simulink model "Simulacion_Discretizada"  (R2020a)
settings: Solver=ode15s  StartTime=0.0  StopTime=20  MaxStep=1e-5  RelTol=1e-3
values from neighbouring files (symbols this model uses):
  alpha_cu = 3.9e-3    (= 0.0039)    [AnalisisDeEstabilidad.m]    (also in LTI_vs_LPV_vs_NL_realimentado.m; Modelo_linealizado.m)
  b_eq = b_m + b_l/(r^2)    (= 2.19444444444e-05)    [LTI_vs_LPV_vs_NL_realimentado.m]    (also in Modelo_linealizado.m)
  ba = 1    [parametros.m]
  C_ts = 0.818    [LTI_vs_LPV_vs_NL_realimentado.m]    (also in Modelo_linealizado.m)
  J_eq = J_m + J_l/(r^2)    (= 1.97847222222e-05)    [LTI_vs_LPV_vs_NL_realimentado.m]    (also in Modelo_linealizado.m)
  Ksa = 1    [parametros.m]
  L_d = 6.6/1000    (= 0.0066)    [Curvas_carc.m]    (also in LTI_vs_LPV_vs_NL_realimentado.m; Modelo_linealizado.m)
  L_ls = 0.8/1000    (= 0.0008)    [LTI_vs_LPV_vs_NL_realimentado.m]    (also in Modelo_linealizado.m)
  L_q = 5.8/1000    (= 0.0058)    [Curvas_carc.m]    (also in LTI_vs_LPV_vs_NL_realimentado.m; Modelo_linealizado.m)
  lambda_m = 0.01546    [Curvas_carc.m]    (also in LTI_vs_LPV_vs_NL_realimentado.m = 0.016; Modelo_linealizado.m = 0.016)
  P_p = 3    [Curvas_carc.m]    (also in LTI_vs_LPV_vs_NL_realimentado.m)
  r = 120    [AnalisisDeEstabilidad.m]    (also in LTI_vs_LPV_vs_NL_realimentado.m; Modelo_linealizado.m; parametros.m)
  R_sREF = R_sref    (= 1.02)    [LTI_vs_LPV_vs_NL_realimentado.m]
  R_ts_amb = 146.7    [LTI_vs_LPV_vs_NL_realimentado.m]    (also in Modelo_linealizado.m)
  Rdp = 3    [parametros.m]
  Rqp = 2    [parametros.m]
  sol = inv(A)*B    [Consigna_de_pos.m]
  sol2 = inv(A)*B    [Consigna_de_pos.m]
  T_amb = T_amb_o    (= 25)    [LTI_vs_LPV_vs_NL_realimentado.m]
  T_sREF = T_sref    (= 40)    [LTI_vs_LPV_vs_NL_realimentado.m]
undefined symbols (not defined in the file or in its folder): K_l, Ke_i, Ke_omega, Ke_theta, Ksia, sigbuilder_block, tau, Ts, V_max, w_n_i, w_n_pos, w_n_v, zit_i, zit_pos, zit_v
libraries: simulink x2
settings Model: Creator=matie  LastModifiedBy=matie

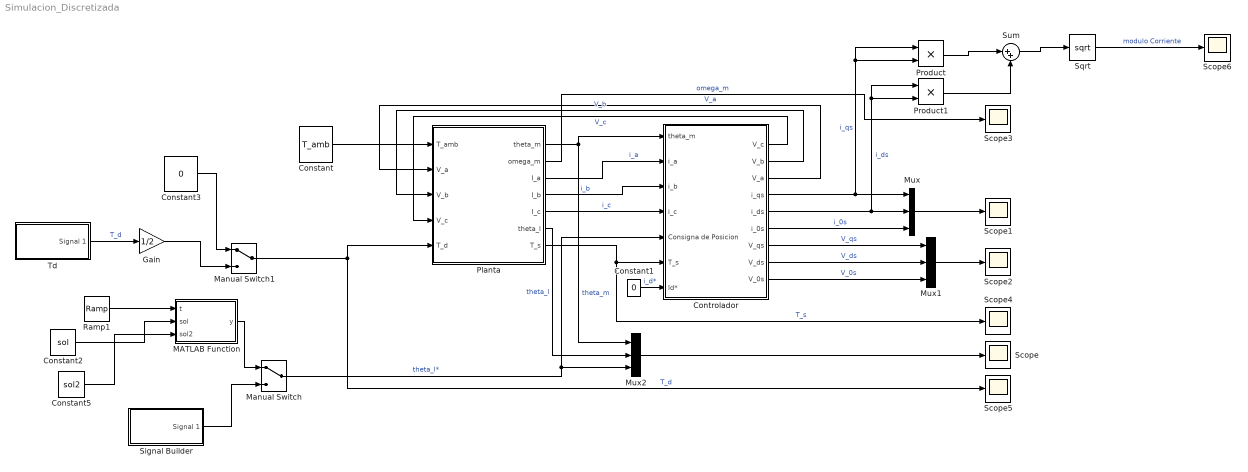
== system Simulacion_Discretizada ==
  Constant : Constant  Value=T_amb  VectorParams1D=off  SampleTime=-1
  Constant1 : Constant  Value=0
  Constant2 : Constant  Value=sol  VectorParams1D=off
  Constant3 : Constant  Value=0  VectorParams1D=off  SampleTime=-1
  Constant5 : Constant  Value=sol2  VectorParams1D=off
  Controlador : Subsystem
  Gain : Gain  Gain=1/2
  MATLAB Function : MATLAB Function  TreatAsAtomicUnit=on
  Manual Switch : ManualSwitch
  Manual Switch1 : ManualSwitch
  Mux : Mux  Inputs=3
  Mux1 : Mux  Inputs=3
  Mux2 : Mux  Inputs=3
  Planta : Subsystem
  Product : Product
  Product1 : Product
  Ramp1 : simulink/Sources/Ramp  slope=1  start=0  InitialOutput=0
  Scope{,1..6} (7 alike) : Scope
  Signal Builder : Subsystem  Tag=STV Subsys  LoadFcn=sigbuilder_block('load');  StartFcn=sigbuilder_block('start');  StopFcn=sigbuilder_block('stop');  ClipboardFcn=sigbuilder_block('clipboard');  mask(Sigbuilder block){tuvar=[0:10]}
      mask help: Simulink:masks:SigbuilderBlock_MD
      mask init:
      | if ~strcmp(get_param(bdroot(gcbh),'SimulationStatus'),'stopped') tuvar = sigbuilder_block('maskInit'); end
      settings: CopyFcn=sigbuilder_block('copy');  DeleteFcn=sigbuilder_block('delete');  ModelCloseFcn=sigbuilder_block('modelClose');  PreSaveFcn=sigbuilder_block('preSave');  PauseFcn=sigbuilder_block('pause');  ContinueFcn=sigbuilder_block('continue');  NameChangeFcn=sigbuilder_block('namechange');  OpenFcn=sigbuilder_block('open',[437.6 199.2 550.4 400 ]);  CloseFcn=sigbuilder_block('close');
      mask Display: plot(0, 0, 100, 100,[2, 2, 32, 32, 2], [68, 8, 8, 68, 68],[32, 2], [38, 38], [32, 19, 2],[53, 60, 44], [32, 17, 17, 2],[16, 16, 31, 31]);txt = getActiveGroup(gcbh);text(2, 100, txt,'verticalAlignment', 'top');
  Sqrt : Sqrt  SaturateOnIntegerOverflow=on
  Sum : Sum  Inputs=|++
  Td : Subsystem  Tag=STV Subsys  LoadFcn=sigbuilder_block('load');  StartFcn=sigbuilder_block('start');  StopFcn=sigbuilder_block('stop');  ClipboardFcn=sigbuilder_block('clipboard');  mask(Sigbuilder block){tuvar=[0:10]}
      mask help: Simulink:masks:SigbuilderBlock_MD
      mask init:
      | if ~strcmp(get_param(bdroot(gcbh),'SimulationStatus'),'stopped') tuvar = sigbuilder_block('maskInit'); end
      settings: CopyFcn=sigbuilder_block('copy');  DeleteFcn=sigbuilder_block('delete');  ModelCloseFcn=sigbuilder_block('modelClose');  PreSaveFcn=sigbuilder_block('preSave');  PauseFcn=sigbuilder_block('pause');  ContinueFcn=sigbuilder_block('continue');  NameChangeFcn=sigbuilder_block('namechange');  OpenFcn=sigbuilder_block('open',[437.6 199.2 550.4 400 ]);  CloseFcn=sigbuilder_block('close');
      mask Display: plot(0, 0, 100, 100,[2, 2, 32, 32, 2], [68, 8, 8, 68, 68],[32, 2], [38, 38], [32, 19, 2],[53, 60, 44], [32, 17, 17, 2],[16, 16, 31, 31]);txt = getActiveGroup(gcbh);text(2, 100, txt,'verticalAlignment', 'top');
  wires:
  Constant/1 -> Planta/1(T_amb)
  Planta/1(theta_m) -> Controlador/1(theta_m), Mux2/1  "theta_m"
  Planta/2(omega_m) -> Scope3/1  "omega_m"
  Planta/3(I_a) -> Controlador/2(i_a)  "i_a"
  Planta/4(I_b) -> Controlador/3(i_b)  "i_b"
  Planta/5(I_c) -> Controlador/4(i_c)  "i_c"
  Controlador/1(V_c) -> Planta/4(V_c)  "V_c"
  Controlador/2(V_b) -> Planta/3(V_b)  "V_b"
  Controlador/3(V_a) -> Planta/2(V_a)  "V_a"
  Constant1/1 -> Controlador/7(Id*)  "i_d*"
  Planta/7(T_s) -> Scope4/1, Controlador/6(T_s)  "T_s"
  Controlador/4(i_qs) -> Product/2, Product/1, Mux/1  "i_qs"
  Controlador/5(i_ds) -> Product1/2, Product1/1, Mux/2  "i_ds"
  Controlador/6(i_0s) -> Mux/3  "i_0s"
  Controlador/7(V_qs) -> Mux1/1  "V_qs"
  Controlador/8(V_ds) -> Mux1/2  "V_ds"
  Controlador/9(V_0s) -> Mux1/3  "V_0s"
  Planta/6(theta_l) -> Mux2/2  "theta_l"
  Manual Switch1/1 -> Planta/5(T_d), Scope5/1  "T_d"
  Manual Switch/1 -> Controlador/5(Consigna de Posicion), Mux2/3  "theta_l*"
  Mux2/1 -> Scope/1
  Mux/1 -> Scope1/1
  Mux1/1 -> Scope2/1
  Constant5/1 -> MATLAB Function/3(sol2)
  Ramp1/1 -> MATLAB Function/1(t)
  Constant2/1 -> MATLAB Function/2(sol)
  MATLAB Function/1(y) -> Manual Switch/1
  Signal Builder/1(Signal 1) -> Manual Switch/2
  Td/1(Signal 1) -> Gain/1  "T_d"
  Constant3/1 -> Manual Switch1/1
  Product/1 -> Sum/1
  Product1/1 -> Sum/2
  Sum/1 -> Sqrt/1
  Sqrt/1 -> Scope6/1  "modulo Corriente"
  Gain/1 -> Manual Switch1/2

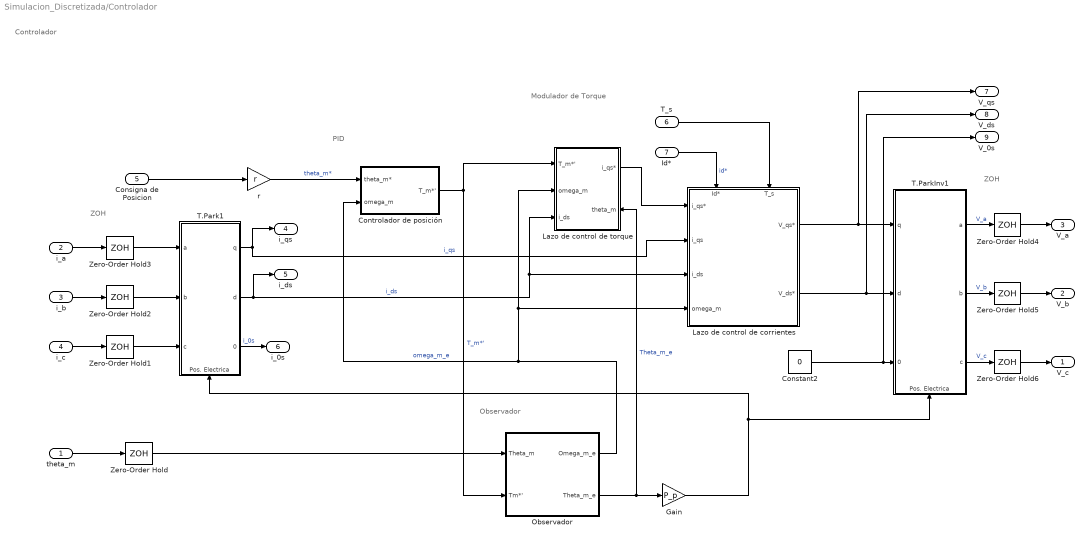
== system Simulacion_Discretizada/Controlador ==
  note: ZOH
  note: ZOH
  note: Observador
  note: Controlador
  note: PID
  note: Modulador de Torque
  theta_m : Inport
  i_a : Inport  Port=2
  i_b : Inport  Port=3
  i_c : Inport  Port=4
  Consigna de Posicion : Inport  Port=5
  T_s : Inport  Port=6
  Id* : Inport  Port=7
  Constant2 : Constant  Value=0
  Controlador de posición : Subsystem
  Gain : Gain  Gain=P_p
  Lazo de control de corrientes : Subsystem
      settings: PortSchema="{\"entries\":[{\"content\":{\"sides\":[{\"content\":{\"connectorIds\":[\"In1\",\"In2\",\"In3\",\"In4\"]},\"type\":\"ConnectorPlacement.EquallySpacedRectSide\",\"uuid\":\"8590a798-b272-4dda-94d3-b02bfe7981cd\"},{\"content\":{\"connectorIds\":[\"Out1\",\"Out2\"],\"side\":\"RIGHT\"},\"type\":\"ConnectorPlacement.EquallySpacedRectSide\",\"uuid\":\"79f7ba4f-ca3d-417b-a956-e8ff79666446\"},{\"content\":{\"connectorIds\":[\"In5\",\"In6\"],\"side\":\"TOP\"},\"type\":\"ConnectorPlacement.EquallySpacedRectSide\",\"uuid\":\"c783970f-a0cd-49ae-b0d9-9eb7b782510c\"}]},\"type\":\"ConnectorPlacement.EquallySpacedConnector\",\"uuid\":\"7f007081-b507-4644-8a4e-ff370ccc3754\"}],\"packageUris\":[\"http://schema.mathworks.com/mf0/Connector/19700101\"],\"version\":\"1.0\"}"
  Lazo de control de torque : Subsystem
      settings: PortSchema="{\"entries\":[{\"content\":{\"sides\":[{\"content\":{\"connectorIds\":[\"In1\",\"In2\",\"In3\"]},\"type\":\"ConnectorPlacement.EquallySpacedRectSide\",\"uuid\":\"ab0e8616-8d3e-4cd7-8423-bd93729455f6\"},{\"content\":{\"connectorIds\":[\"Out1\",\"In4\"],\"side\":\"RIGHT\"},\"type\":\"ConnectorPlacement.EquallySpacedRectSide\",\"uuid\":\"bacb25e2-23a7-49b0-9cd8-46522174ac61\"},{\"content\":{\"connectorIds\":[],\"side\":\"TOP\"},\"type\":\"ConnectorPlacement.EquallySpacedRectSide\",\"uuid\":\"92980fe9-d82b-422b-ba0e-4e399ce43552\"},{\"content\":{\"connectorIds\":[],\"side\":\"BOTTOM\"},\"type\":\"ConnectorPlacement.EquallySpacedRectSide\",\"uuid\":\"d03b3e30-9585-41dd-826f-10e3a5c14235\"}]},\"type\":\"ConnectorPlacement.EquallySpacedConnector\",\"uuid\":\"7c3e8c07-5c99-45fd-a37d-868b0a52132c\"}],\"packageUris\":[\"http://schema.mathworks.com/mf0/Connector/19700101\"],\"version\":\"1.0\"}"
  Observador : Subsystem
  T.Park1 : Subsystem
      settings: PortSchema="{\"entries\":[{\"content\":{\"sides\":[{\"content\":{\"connectorIds\":[\"In1\",\"In2\",\"In3\"]},\"type\":\"ConnectorPlacement.EquallySpacedRectSide\",\"uuid\":\"2bfbe7ef-652a-4797-b13c-b84c243bd68c\"},{\"content\":{\"connectorIds\":[\"Out1\",\"Out2\",\"Out3\"],\"side\":\"RIGHT\"},\"type\":\"ConnectorPlacement.EquallySpacedRectSide\",\"uuid\":\"075def0e-c436-44dc-ba25-82cf6ffae869\"},{\"content\":{\"connectorIds\":[\"In4\"],\"side\":\"TOP\"},\"type\":\"ConnectorPlacement.EquallySpacedRectSide\",\"uuid\":\"95d81334-e332-4f04-a2cb-c4692f91809c\"},{\"content\":{\"connectorIds\":[],\"side\":\"BOTTOM\"},\"type\":\"ConnectorPlacement.EquallySpacedRectSide\",\"uuid\":\"85b95360-e43d-49d1-a18f-690334b045e6\"}]},\"type\":\"ConnectorPlacement.EquallySpacedConnector\",\"uuid\":\"b90f9cad-0277-459c-bcac-17172872a787\"}],\"packageUris\":[\"http://schema.mathworks.com/mf0/Connector/19700101\"],\"version\":\"1.0\"}"
  T.ParkInv1 : Subsystem
      settings: PortSchema="{\"entries\":[{\"content\":{\"sides\":[{\"content\":{\"connectorIds\":[\"In1\",\"In2\",\"In3\"]},\"type\":\"ConnectorPlacement.EquallySpacedRectSide\",\"uuid\":\"aef3590a-5fc0-4a95-8f41-1fc79c0f3fe7\"},{\"content\":{\"connectorIds\":[\"Out1\",\"Out2\",\"Out3\"],\"side\":\"RIGHT\"},\"type\":\"ConnectorPlacement.EquallySpacedRectSide\",\"uuid\":\"4e7c387b-9bca-48cc-a151-2357bd6b7b1d\"},{\"content\":{\"connectorIds\":[],\"side\":\"TOP\"},\"type\":\"ConnectorPlacement.EquallySpacedRectSide\",\"uuid\":\"1231932f-f9d3-49e6-b404-2af91cb220c6\"},{\"content\":{\"connectorIds\":[\"In4\"],\"side\":\"BOTTOM\"},\"type\":\"ConnectorPlacement.EquallySpacedRectSide\",\"uuid\":\"5c8d0cfe-c367-499e-bd37-95f7c8af20a1\"}]},\"type\":\"ConnectorPlacement.EquallySpacedConnector\",\"uuid\":\"48e39a78-817d-4753-b518-4d689d2c1635\"}],\"packageUris\":[\"http://schema.mathworks.com/mf0/Connector/19700101\"],\"version\":\"1.0\"}"
  Zero-Order Hold{,1..6} (7 alike) : ZeroOrderHold  SampleTime=Ts
  r : Gain  Gain=r
  V_c : Outport
  V_b : Outport  Port=2
  V_a : Outport  Port=3
  i_qs : Outport  Port=4
  i_ds : Outport  Port=5
  i_0s : Outport  Port=6
  V_qs : Outport  Port=7
  V_ds : Outport  Port=8
  V_0s : Outport  Port=9
  wires:
  i_b/1 -> Zero-Order Hold2/1
  i_a/1 -> Zero-Order Hold3/1
  i_c/1 -> Zero-Order Hold1/1
  T.Park1/1(0) -> i_0s/1  "i_0s"
  T.Park1/2(d) -> Lazo de control de torque/3(i_ds), Lazo de control de corrientes/3(i_ds), i_ds/1  "i_ds"
  T_s/1 -> Lazo de control de corrientes/6(T_s)
  Observador/1(Omega_m_e) -> Controlador de posición/2(omega_m), Lazo de control de torque/2(omega_m), Lazo de control de corrientes/4(omega_m)  "omega_m_e"
  T.Park1/3(q) -> i_qs/1, Lazo de control de corrientes/2(i_qs)  "i_qs"
  Gain/1 -> T.Park1/4(Pos. Electrica), T.ParkInv1/4(Pos. Electrica)
  Controlador de posición/1(T_m*') -> Lazo de control de torque/1(T_m*'), Observador/2(Tm*')  "T_m*'"
  Consigna de Posicion/1 -> r/1
  T.ParkInv1/3(c) -> Zero-Order Hold6/1  "V_c"
  T.ParkInv1/2(b) -> Zero-Order Hold5/1  "V_b"
  T.ParkInv1/1(a) -> Zero-Order Hold4/1  "V_a"
  Constant2/1 -> V_0s/1, T.ParkInv1/3(0)
  theta_m/1 -> Zero-Order Hold/1
  Observador/2(Theta_m_e) -> Gain/1, Lazo de control de torque/4(theta_m)  "Theta_m_e"
  Lazo de control de corrientes/2(V_ds*) -> V_ds/1, T.ParkInv1/2(d)
  Lazo de control de corrientes/1(V_qs*) -> V_qs/1, T.ParkInv1/1(q)
  Lazo de control de torque/1(i_qs*) -> Lazo de control de corrientes/1(i_qs*)
  Id*/1 -> Lazo de control de corrientes/5(Id*)  "id*"
  r/1 -> Controlador de posición/1(theta_m*)  "theta_m*"
  Zero-Order Hold/1 -> Observador/1(Theta_m)
  Zero-Order Hold1/1 -> T.Park1/1(c)
  Zero-Order Hold2/1 -> T.Park1/2(b)
  Zero-Order Hold3/1 -> T.Park1/3(a)
  Zero-Order Hold4/1 -> V_a/1
  Zero-Order Hold5/1 -> V_b/1
  Zero-Order Hold6/1 -> V_c/1

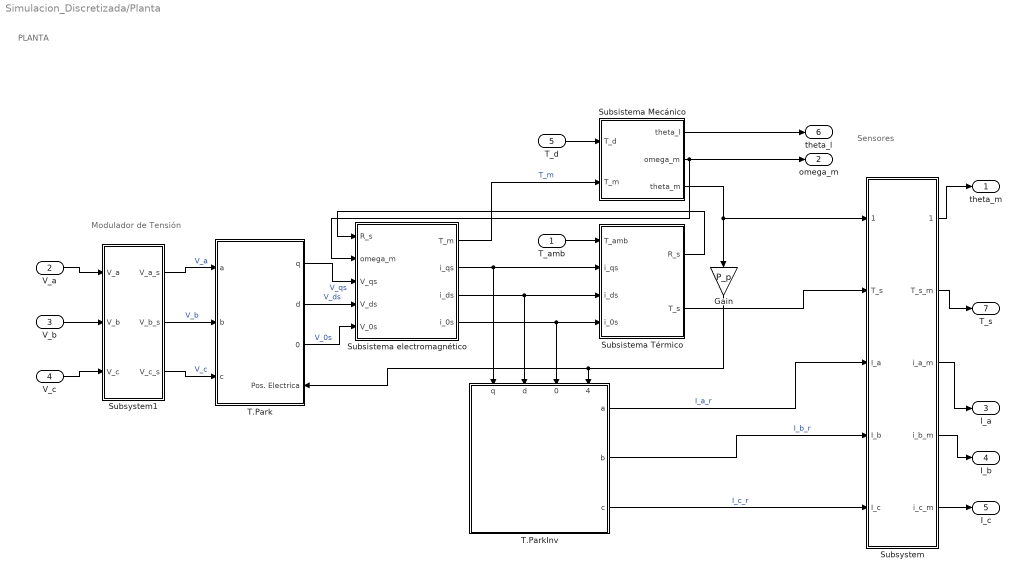
== system Simulacion_Discretizada/Planta ==
  note: PLANTA
  note: Sensores
  note: Modulador de
      | Tensión
  T_amb : Inport
  V_a : Inport  Port=2
  V_b : Inport  Port=3
  V_c : Inport  Port=4
  T_d : Inport  Port=5
  "\tSubsistema Térmico" : Subsystem
  Gain : Gain  Gain=P_p
  Subsistema Mecánico : Subsystem
  Subsistema electromagnético : Subsystem
  Subsystem : Subsystem
  Subsystem1 : Subsystem
  T.Park : Subsystem
      settings: PortSchema="{\"entries\":[{\"content\":{\"sides\":[{\"content\":{\"connectorIds\":[\"In1\",\"In2\",\"In3\"]},\"type\":\"ConnectorPlacement.EquallySpacedRectSide\",\"uuid\":\"2bfbe7ef-652a-4797-b13c-b84c243bd68c\"},{\"content\":{\"connectorIds\":[\"Out1\",\"Out2\",\"Out3\",\"In4\"],\"side\":\"RIGHT\"},\"type\":\"ConnectorPlacement.EquallySpacedRectSide\",\"uuid\":\"075def0e-c436-44dc-ba25-82cf6ffae869\"},{\"content\":{\"connectorIds\":[],\"side\":\"TOP\"},\"type\":\"ConnectorPlacement.EquallySpacedRectSide\",\"uuid\":\"95d81334-e332-4f04-a2cb-c4692f91809c\"}]},\"type\":\"ConnectorPlacement.EquallySpacedConnector\",\"uuid\":\"b90f9cad-0277-459c-bcac-17172872a787\"}],\"packageUris\":[\"http://schema.mathworks.com/mf0/Connector/19700101\"],\"version\":\"1.0\"}"
  T.ParkInv : Subsystem
      settings: PortSchema="{\"entries\":[{\"content\":{\"sides\":[{\"content\":{\"connectorIds\":[\"In1\",\"In2\",\"In3\",\"In4\"]},\"type\":\"ConnectorPlacement.EquallySpacedRectSide\",\"uuid\":\"aef3590a-5fc0-4a95-8f41-1fc79c0f3fe7\"},{\"content\":{\"connectorIds\":[],\"side\":\"RIGHT\"},\"type\":\"ConnectorPlacement.EquallySpacedRectSide\",\"uuid\":\"4e7c387b-9bca-48cc-a151-2357bd6b7b1d\"},{\"content\":{\"connectorIds\":[],\"side\":\"TOP\"},\"type\":\"ConnectorPlacement.EquallySpacedRectSide\",\"uuid\":\"1231932f-f9d3-49e6-b404-2af91cb220c6\"},{\"content\":{\"connectorIds\":[\"Out1\",\"Out2\",\"Out3\"],\"side\":\"BOTTOM\"},\"type\":\"ConnectorPlacement.EquallySpacedRectSide\",\"uuid\":\"4f29e626-7677-496e-bb82-59a3ecbc7a95\"}]},\"type\":\"ConnectorPlacement.EquallySpacedConnector\",\"uuid\":\"48e39a78-817d-4753-b518-4d689d2c1635\"}],\"packageUris\":[\"http://schema.mathworks.com/mf0/Connector/19700101\"],\"version\":\"1.0\"}"
  theta_m : Outport
  omega_m : Outport  Port=2
  I_a : Outport  Port=3
  I_b : Outport  Port=4
  I_c : Outport  Port=5
  theta_l : Outport  Port=6
  T_s : Outport  Port=7
  wires:
  Subsistema Mecánico/3(theta_m) -> Subsystem/1(theta_m), Gain/1
  Gain/1 -> T.Park/4(Pos. Electrica), T.ParkInv/4(Pos. Electrica)
  T.Park/1(q) -> Subsistema electromagnético/3(V_qs)  "V_qs"
  Subsistema Mecánico/2(omega_m) -> Subsistema electromagnético/2(omega_m), omega_m/1
  Subsistema electromagnético/2(i_qs) -> "\tSubsistema Térmico"/2(i_qs), T.ParkInv/1(q)
  Subsistema electromagnético/1(T_m) -> Subsistema Mecánico/2(T_m)  "T_m"
  Subsistema electromagnético/4(i_0s) -> "\tSubsistema Térmico"/4(i_0s), T.ParkInv/3(0)
  Subsistema electromagnético/3(i_ds) -> "\tSubsistema Térmico"/3(i_ds), T.ParkInv/2(d)
  Subsistema Mecánico/1(theta_l) -> theta_l/1
  T.Park/3(0) -> Subsistema electromagnético/5(V_0s)  "V_0s"
  T.Park/2(d) -> Subsistema electromagnético/4(V_ds)  "V_ds"
  T_d/1 -> Subsistema Mecánico/1(T_d)
  T_amb/1 -> "\tSubsistema Térmico"/1(T_amb)
  "\tSubsistema Térmico"/1(R_s) -> Subsistema electromagnético/1(R_s)
  "\tSubsistema Térmico"/2(T_s) -> Subsystem/2(T_s)
  T.ParkInv/1(a) -> Subsystem/3(I_a)  "I_a_r"
  T.ParkInv/2(b) -> Subsystem/4(I_b)  "I_b_r"
  T.ParkInv/3(c) -> Subsystem/5(I_c)  "I_c_r"
  Subsystem/1(theta_m_m) -> theta_m/1
  Subsystem/2(T_s_m) -> T_s/1
  Subsystem/3(i_a_m) -> I_a/1
  Subsystem/4(i_b_m) -> I_b/1
  Subsystem/5(i_c_m) -> I_c/1
  V_a/1 -> Subsystem1/1(V_a)
  V_b/1 -> Subsystem1/2(V_b)
  V_c/1 -> Subsystem1/3(V_c)
  Subsystem1/1(V_a_s) -> T.Park/1(a)  "V_a"
  Subsystem1/2(V_b_s) -> T.Park/2(b)  "V_b"
  Subsystem1/3(V_c_s) -> T.Park/3(c)  "V_c"

== system Simulacion_Discretizada/Signal Builder ==
  Demux : Demux  Tag=STV Demux  Outputs=1
      settings: DisplayOption=none
  FromWs : FromWorkspace  Tag=STV FromWs  VariableName=tuvar
      SigBuilderData=|
      | common.afterFinalStr = 'Extrapolate'
      | common.sampleTime = 0
      | dataSet.timeRange = [0 20]
      | dataSet.name = 'Group 1'
      | sbobj.Groups.Name = 'Group 1'
      | sbobj.Groups.Signals.Name = 'Signal 1'
      | sbobj.Groups.Signals.XData = [0 1 6 11 16 20]
      | sbobj.Groups.Signals.YData = [0 0 6.28318530718 6.28318530718 0 0]
      | sbobj.Groups.TimeRange = [0 20]
  Signal 1 : Outport  Tag=STV Outport
  wires:
  Demux/1 -> Signal 1/1
  FromWs/1 -> Demux/1

== system Simulacion_Discretizada/Td ==
  Demux : Demux  Tag=STV Demux  Outputs=1
      settings: DisplayOption=none
  FromWs : FromWorkspace  Tag=STV FromWs  VariableName=tuvar
      SigBuilderData=|
      | common.afterFinalStr = 'Extrapolate'
      | common.sampleTime = 0
      | dataSet.timeRange = [0 20]
      | dataSet.name = 'Group 1'
      | sbobj.Groups.Name = 'Group 1'
      | sbobj.Groups.Signals.Name = 'Signal 1'
      | sbobj.Groups.Signals.XData = [0 6.5 6.5 8.5 8.5 10.5 10.5 20]
      | sbobj.Groups.Signals.YData = [0 0 5 5 -5 -5 0 0]
      | sbobj.Groups.TimeRange = [0 20]
  Signal 1 : Outport  Tag=STV Outport
  wires:
  Demux/1 -> Signal 1/1
  FromWs/1 -> Demux/1

== system Simulacion_Discretizada/Controlador/Controlador de posición ==
  theta_m* : Inport
  omega_m : Inport  Port=2
  Constant2 : Constant  Value=sol  VectorParams1D=off
  Constant5 : Constant  Value=sol2  VectorParams1D=off
  Derivative : Derivative  CoefficientInTFapproximation=0
  Gain : Gain  Gain=r
  Manual Switch : ManualSwitch
  Ramp : simulink/Sources/Ramp  slope=1  start=0  InitialOutput=0
  Subsystem : Subsystem
  consigna_velocidad : MATLAB Function  TreatAsAtomicUnit=on
  T_m*' : Outport
  wires:
  theta_m*/1 -> Derivative/1
  Constant5/1 -> consigna_velocidad/3(sol2)
  Constant2/1 -> consigna_velocidad/2(sol)
  Derivative/1 -> Manual Switch/2  "omega_m*"
  consigna_velocidad/1(y) -> Gain/1
  Gain/1 -> Manual Switch/1
  Ramp/1 -> consigna_velocidad/1(t)
  Manual Switch/1 -> Subsystem/1(omega_m*)  "omega_m*"
  omega_m/1 -> Subsystem/2(omega_m)
  Subsystem/1(T_m*') -> T_m*'/1

== system Simulacion_Discretizada/Controlador/Lazo de control de corrientes ==
  i_qs* : Inport
  i_qs : Inport  Port=2
  i_ds : Inport  Port=3
  omega_m : Inport  Port=4
  Id* : Inport  Port=5
  T_s : Inport  Port=6
  Control de I_ds : Subsystem
      settings: PortSchema="{\"entries\":[{\"content\":{\"sides\":[{\"content\":{\"connectorIds\":[\"In1\",\"In2\",\"In3\",\"In4\"]},\"type\":\"ConnectorPlacement.EquallySpacedRectSide\",\"uuid\":\"ffce1851-57e2-41df-aed0-a87e2179134d\"},{\"content\":{\"connectorIds\":[\"Out1\"],\"side\":\"RIGHT\"},\"type\":\"ConnectorPlacement.EquallySpacedRectSide\",\"uuid\":\"747f8c9d-35f1-4917-b439-3fa2ce1f796d\"},{\"content\":{\"connectorIds\":[],\"side\":\"TOP\"},\"type\":\"ConnectorPlacement.EquallySpacedRectSide\",\"uuid\":\"8177f07d-0fa6-4905-a4da-67659c71ef29\"},{\"content\":{\"connectorIds\":[\"In5\"],\"side\":\"BOTTOM\"},\"type\":\"ConnectorPlacement.EquallySpacedRectSide\",\"uuid\":\"6dd9ac8a-27c9-4038-bd4e-8ef4f6a79f96\"}]},\"type\":\"ConnectorPlacement.EquallySpacedConnector\",\"uuid\":\"e8499173-6965-4bf7-863b-b1df3b035aa5\"}],\"packageUris\":[\"http://schema.mathworks.com/mf0/Connector/19700101\"],\"version\":\"1.0\"}"
  Control de I_qs : Subsystem
      settings: PortSchema="{\"entries\":[{\"content\":{\"sides\":[{\"content\":{\"connectorIds\":[\"In1\",\"In2\",\"In3\",\"In4\"]},\"type\":\"ConnectorPlacement.EquallySpacedRectSide\",\"uuid\":\"ffce1851-57e2-41df-aed0-a87e2179134d\"},{\"content\":{\"connectorIds\":[\"Out1\"],\"side\":\"RIGHT\"},\"type\":\"ConnectorPlacement.EquallySpacedRectSide\",\"uuid\":\"747f8c9d-35f1-4917-b439-3fa2ce1f796d\"},{\"content\":{\"connectorIds\":[\"In5\"],\"side\":\"TOP\"},\"type\":\"ConnectorPlacement.EquallySpacedRectSide\",\"uuid\":\"8177f07d-0fa6-4905-a4da-67659c71ef29\"}]},\"type\":\"ConnectorPlacement.EquallySpacedConnector\",\"uuid\":\"e8499173-6965-4bf7-863b-b1df3b035aa5\"}],\"packageUris\":[\"http://schema.mathworks.com/mf0/Connector/19700101\"],\"version\":\"1.0\"}"
  Evolución R_s : Subsystem
  Gain10 : Gain  Gain=P_p
  V_qs* : Outport
  V_ds* : Outport  Port=2
  wires:
  Gain10/1 -> Control de I_qs/1(omega_e), Control de I_ds/4(omega_e)
  i_qs*/1 -> Control de I_qs/5(i_qs*)
  i_ds/1 -> Control de I_qs/3(i_ds), Control de I_ds/1(i_ds)
  Control de I_qs/1(V_qs*) -> V_qs*/1
  i_qs/1 -> Control de I_qs/4(i_qs), Control de I_ds/2(i_qs)
  T_s/1 -> Evolución R_s/1(T_s)
  Control de I_ds/1(V_ds*) -> V_ds*/1
  omega_m/1 -> Gain10/1
  Id*/1 -> Control de I_ds/5(i_ds*)
  Evolución R_s/1(R_s) -> Control de I_ds/3(R_s), Control de I_qs/2(R_s)

== system Simulacion_Discretizada/Controlador/Lazo de control de torque ==
  note: Linealización por realimentación no lineal
  note: T_m*
  T_m*' : Inport
  omega_m : Inport  Port=2
  i_ds : Inport  Port=3
  theta_m : Inport  Port=4
  1/r : Gain  Gain=1/r
  Constant3 : Constant  Value=lambda_m
  Divide : Product  Inputs=*/
  Gain3 : Gain  Gain=b_eq
  Gain4 : Gain  Gain=L_d-L_q
  Gain5 : Gain  Gain=3*P_p/2
  Kl/r : Gain  Gain=K_l/r
  Sum11 : Sum  Inputs=|+++
  Sum12 : Sum  Inputs=|++
  Trigonometric Function2 : Trigonometry
  i_qs* : Outport
  wires:
  i_ds/1 -> Gain4/1
  Gain4/1 -> Sum12/2
  Gain3/1 -> Sum11/3
  omega_m/1 -> Gain3/1
  Sum11/1 -> Divide/1  "T_m*"
  Constant3/1 -> Sum12/1
  Gain5/1 -> Divide/2
  Sum12/1 -> Gain5/1
  Divide/1 -> i_qs*/1  "i_qs*"
  T_m*'/1 -> Sum11/2
  Trigonometric Function2/1 -> Kl/r/1
  1/r/1 -> Trigonometric Function2/1
  Kl/r/1 -> Sum11/1
  theta_m/1 -> 1/r/1

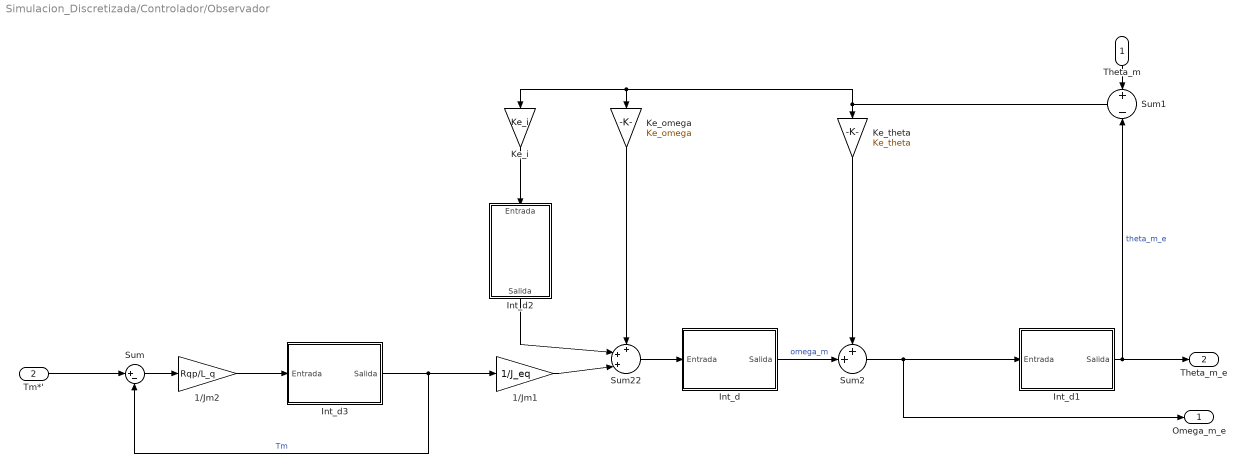
== system Simulacion_Discretizada/Controlador/Observador ==
  Theta_m : Inport
  Tm*' : Inport  Port=2
  1/Jm1 : Gain  Gain=1/J_eq
  1/Jm2 : Gain  Gain=Rqp/L_q
  Int_d : Subsystem
  Int_d1 : Subsystem
  Int_d2 : Subsystem
  Int_d3 : Subsystem
  Ke_i : Gain  Gain=Ke_i
  Ke_omega : Gain  Gain=Ke_omega
  Ke_theta : Gain  Gain=Ke_theta
  Sum : Sum  Inputs=|+-
  Sum1 : Sum  Inputs=+-
  Sum2 : Sum  Inputs=++|
  Sum22 : Sum  Inputs=+++|
  Omega_m_e : Outport
  Theta_m_e : Outport  Port=2
  wires:
  Ke_omega/1 -> Sum22/1
  Sum2/1 -> Int_d1/1(Entrada), Omega_m_e/1
  Ke_theta/1 -> Sum2/1
  1/Jm1/1 -> Sum22/3
  Theta_m/1 -> Sum1/1
  Tm*'/1 -> Sum/1
  Int_d3/1(Salida) -> 1/Jm1/1, Sum/2  "Tm"
  Int_d2/1(Salida) -> Sum22/2
  Sum1/1 -> Ke_i/1, Ke_omega/1, Ke_theta/1
  Ke_i/1 -> Int_d2/1(Entrada)
  Sum22/1 -> Int_d/1(Entrada)
  Int_d/1(Salida) -> Sum2/2  "omega_m"
  Int_d1/1(Salida) -> Theta_m_e/1, Sum1/2  "theta_m_e"
  Sum/1 -> 1/Jm2/1
  1/Jm2/1 -> Int_d3/1(Entrada)

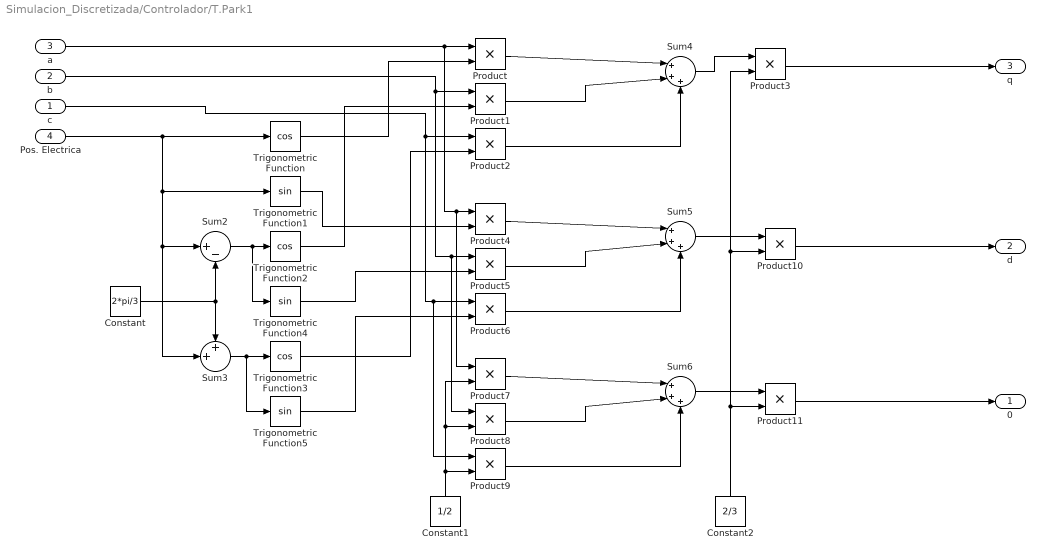
== system Simulacion_Discretizada/Controlador/T.Park1 ==
  c : Inport
  b : Inport  Port=2
  a : Inport  Port=3
  Pos. Electrica : Inport  Port=4
  Constant : Constant  Value=2*pi/3
  Constant1 : Constant  Value=1/2
  Constant2 : Constant  Value=2/3
  Product{,1..11} (12 alike) : Product
  Sum2 : Sum  Inputs=|+-
  Sum3 : Sum  Inputs=++|
  Sum4 : Sum  Inputs=|+++
  Sum5 : Sum  Inputs=|+++
  Sum6 : Sum  Inputs=|+++
  Trigonometric Function : Trigonometry  Operator=cos
  Trigonometric Function1 : Trigonometry
  Trigonometric Function2 : Trigonometry  Operator=cos
  Trigonometric Function3 : Trigonometry  Operator=cos
  Trigonometric Function4 : Trigonometry
  Trigonometric Function5 : Trigonometry
  0 : Outport
  d : Outport  Port=2
  q : Outport  Port=3
  wires:
  Product1/1 -> Sum4/2
  c/1 -> Product9/1, Product6/1, Product2/1
  Constant1/1 -> Product9/2, Product8/2, Product7/2
  Sum2/1 -> Trigonometric Function4/1, Trigonometric Function2/1
  Constant2/1 -> Product11/2, Product10/2, Product3/2
  b/1 -> Product8/1, Product5/1, Product1/1
  Product11/1 -> 0/1
  Pos. Electrica/1 -> Sum3/2, Sum2/1, Trigonometric Function1/1, Trigonometric Function/1
  Trigonometric Function2/1 -> Product1/2
  Trigonometric Function5/1 -> Product6/2
  Product6/1 -> Sum5/3
  Trigonometric Function1/1 -> Product4/2
  Constant/1 -> Sum3/1, Sum2/2
  Sum5/1 -> Product10/1
  Product3/1 -> q/1
  Sum4/1 -> Product3/1
  Trigonometric Function3/1 -> Product2/2
  Trigonometric Function/1 -> Product/2
  a/1 -> Product7/1, Product4/1, Product/1
  Product10/1 -> d/1
  Trigonometric Function4/1 -> Product5/2
  Product/1 -> Sum4/1
  Product7/1 -> Sum6/1
  Sum3/1 -> Trigonometric Function5/1, Trigonometric Function3/1
  Product2/1 -> Sum4/3
  Product9/1 -> Sum6/3
  Product5/1 -> Sum5/2
  Product4/1 -> Sum5/1
  Sum6/1 -> Product11/1
  Product8/1 -> Sum6/2

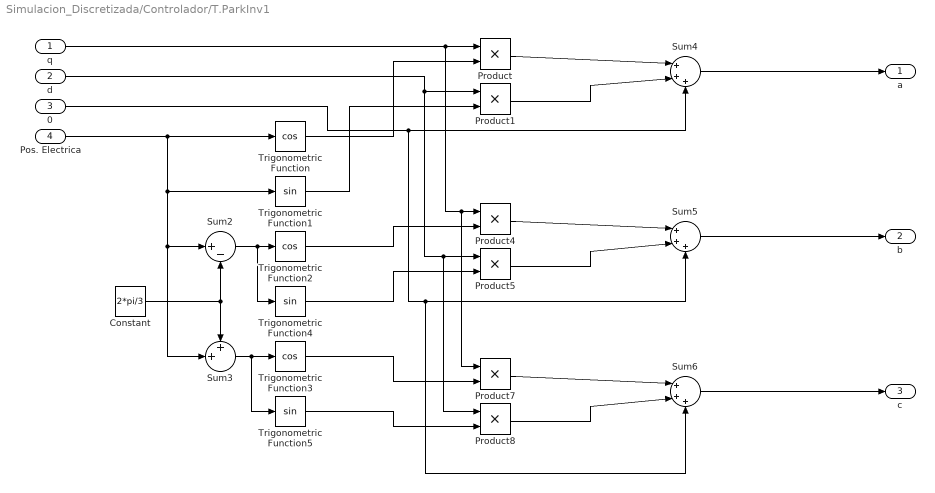
== system Simulacion_Discretizada/Controlador/T.ParkInv1 ==
  q : Inport
  d : Inport  Port=2
  0 : Inport  Port=3
  Pos. Electrica : Inport  Port=4
  Constant : Constant  Value=2*pi/3
  Product{,1,4..5,7..8} (6 alike) : Product
  Sum2 : Sum  Inputs=|+-
  Sum3 : Sum  Inputs=++|
  Sum4 : Sum  Inputs=|+++
  Sum5 : Sum  Inputs=|+++
  Sum6 : Sum  Inputs=|+++
  Trigonometric Function : Trigonometry  Operator=cos
  Trigonometric Function1 : Trigonometry
  Trigonometric Function2 : Trigonometry  Operator=cos
  Trigonometric Function3 : Trigonometry  Operator=cos
  Trigonometric Function4 : Trigonometry
  Trigonometric Function5 : Trigonometry
  a : Outport
  b : Outport  Port=2
  c : Outport  Port=3
  wires:
  Constant/1 -> Sum3/1, Sum2/2
  Pos. Electrica/1 -> Sum3/2, Sum2/1, Trigonometric Function1/1, Trigonometric Function/1
  Trigonometric Function3/1 -> Product7/2
  d/1 -> Product8/1, Product5/1, Product1/1
  0/1 -> Sum4/3, Sum5/3, Sum6/3
  Product8/1 -> Sum6/2
  Product7/1 -> Sum6/1
  q/1 -> Product7/1, Product4/1, Product/1
  Sum3/1 -> Trigonometric Function5/1, Trigonometric Function3/1
  Trigonometric Function5/1 -> Product8/2
  Sum6/1 -> c/1
  Product1/1 -> Sum4/2
  Sum2/1 -> Trigonometric Function4/1, Trigonometric Function2/1
  Sum4/1 -> a/1
  Sum5/1 -> b/1
  Trigonometric Function1/1 -> Product1/2
  Product5/1 -> Sum5/2
  Trigonometric Function2/1 -> Product4/2
  Product4/1 -> Sum5/1
  Product/1 -> Sum4/1
  Trigonometric Function/1 -> Product/2
  Trigonometric Function4/1 -> Product5/2

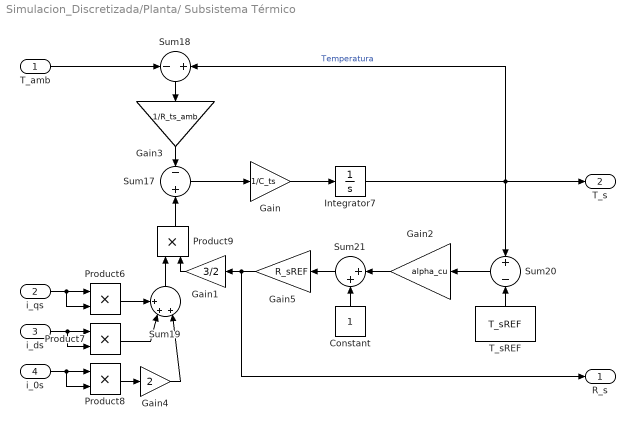
== system Simulacion_Discretizada/Planta/	Subsistema Térmico ==
  T_amb : Inport
  i_qs : Inport  Port=2
  i_ds : Inport  Port=3
  i_0s : Inport  Port=4
  Constant : Constant
  Gain : Gain  Gain=1/C_ts
  Gain1 : Gain  Gain=3/2
  Gain2 : Gain  Gain=alpha_cu
  Gain3 : Gain  Gain=1/R_ts_amb
  Gain4 : Gain  Gain=2
  Gain5 : Gain  Gain=R_sREF
  Integrator7 : Integrator  InitialCondition=T_amb
  Product{6..9} (4 alike) : Product
  Sum17 : Sum  Inputs=-+
  Sum18 : Sum  Inputs=-+
  Sum19 : Sum  Inputs=+++|
  Sum20 : Sum  Inputs=+-
  Sum21 : Sum  Inputs=|++
  T_sREF : Constant  Value=T_sREF
  R_s : Outport
  T_s : Outport  Port=2
  wires:
  Gain4/1 -> Sum19/3
  Integrator7/1 -> Sum18/2, T_s/1, Sum20/1  "Temperatura"
  i_ds/1 -> Product7/2, Product7/1
  Product8/1 -> Gain4/1
  Product7/1 -> Sum19/2
  T_amb/1 -> Sum18/1
  Sum18/1 -> Gain3/1
  Product6/1 -> Sum19/1
  Gain/1 -> Integrator7/1
  Product9/1 -> Sum17/2
  Sum17/1 -> Gain/1
  Gain3/1 -> Sum17/1
  T_sREF/1 -> Sum20/2
  Sum20/1 -> Gain2/1
  Gain1/1 -> Product9/2
  i_qs/1 -> Product6/1, Product6/2
  Sum19/1 -> Product9/1
  Gain2/1 -> Sum21/1
  i_0s/1 -> Product8/2, Product8/1
  Constant/1 -> Sum21/2
  Sum21/1 -> Gain5/1
  Gain5/1 -> R_s/1, Gain1/1

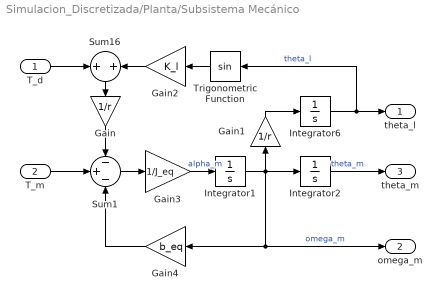
== system Simulacion_Discretizada/Planta/Subsistema Mecánico ==
  T_d : Inport
  T_m : Inport  Port=2
  Gain : Gain  Gain=1/r
  Gain1 : Gain  Gain=1/r
  Gain2 : Gain  Gain=K_l
  Gain3 : Gain  Gain=1/J_eq
  Gain4 : Gain  Gain=b_eq
  Integrator1 : Integrator
  Integrator2 : Integrator
  Integrator6 : Integrator
  Sum1 : Sum  Inputs=-+-
  Sum16 : Sum  Inputs=+|+
  Trigonometric Function : Trigonometry
  theta_l : Outport
  omega_m : Outport  Port=2
  theta_m : Outport  Port=3
  wires:
  Integrator2/1 -> theta_m/1  "theta_m"
  Integrator6/1 -> theta_l/1, Trigonometric Function/1  "theta_l"
  Gain1/1 -> Integrator6/1
  Gain4/1 -> Sum1/3
  T_m/1 -> Sum1/2
  Integrator1/1 -> Gain4/1, omega_m/1, Integrator2/1, Gain1/1  "omega_m"
  Trigonometric Function/1 -> Gain2/1
  Gain2/1 -> Sum16/2
  Sum16/1 -> Gain/1
  Gain/1 -> Sum1/1
  T_d/1 -> Sum16/1
  Sum1/1 -> Gain3/1
  Gain3/1 -> Integrator1/1  "alpha_m"

== system Simulacion_Discretizada/Planta/Subsistema electromagnético ==
  R_s : Inport
  omega_m : Inport  Port=2
  V_qs : Inport  Port=3
  V_ds : Inport  Port=4
  V_0s : Inport  Port=5
  Gain2 : Gain  Gain=L_q
  Gain3 : Gain  Gain=L_d
  Gain4 : Gain  Gain=P_p
  Subsystem : Subsystem
  Subsystem1 : Subsystem
  Subsystem2 : Subsystem
  Subsystem3 : Subsystem
  T_m : Outport
  i_qs : Outport  Port=2
  i_ds : Outport  Port=3
  i_0s : Outport  Port=4
  wires:
  omega_m/1 -> Gain4/1
  Subsystem/1(i_qs) -> i_qs/1, Subsystem3/2(i_qs), Gain2/1
  Subsystem1/1(i_ds) -> i_ds/1, Subsystem3/1(I_ds), Gain3/1
  Gain2/1 -> Subsystem1/1(i_qs*Lq)
  Gain3/1 -> Subsystem/4(i_ds*L_d)
  Gain4/1 -> Subsystem1/2(omega_e), Subsystem/3(omega_e)
  V_qs/1 -> Subsystem/1(V_qs)
  R_s/1 -> Subsystem/2(R_s), Subsystem1/3(R_s), Subsystem2/1(R_s)
  V_ds/1 -> Subsystem1/4(V_ds)
  V_0s/1 -> Subsystem2/2(V_0s)
  Subsystem2/1(i_0s) -> i_0s/1
  Subsystem3/1(T_m) -> T_m/1

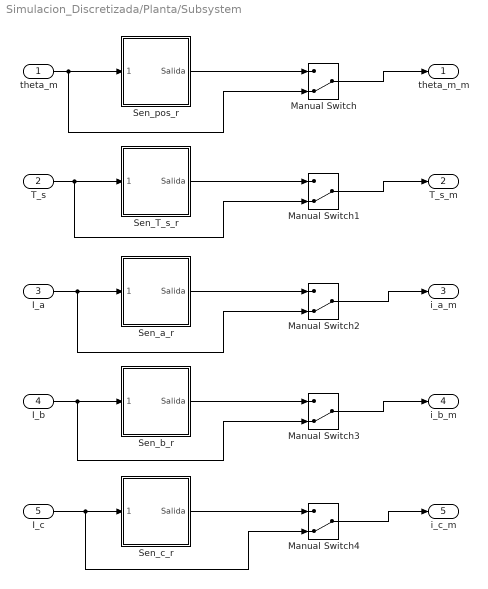
== system Simulacion_Discretizada/Planta/Subsystem ==
  theta_m : Inport
  T_s : Inport  Port=2
  I_a : Inport  Port=3
  I_b : Inport  Port=4
  I_c : Inport  Port=5
  Manual Switch{,1..4} (5 alike) : ManualSwitch  CurrentSetting=0
  Sen_T_s_r : Subsystem
  Sen_a_r : Subsystem
  Sen_b_r : Subsystem
  Sen_c_r : Subsystem
  Sen_pos_r : Subsystem
  theta_m_m : Outport
  T_s_m : Outport  Port=2
  i_a_m : Outport  Port=3
  i_b_m : Outport  Port=4
  i_c_m : Outport  Port=5
  wires:
  I_a/1 -> Manual Switch2/2, Sen_a_r/1(Entrada)
  I_b/1 -> Manual Switch3/2, Sen_b_r/1(Entrada)
  T_s/1 -> Manual Switch1/2, Sen_T_s_r/1(Entrada)
  Manual Switch3/1 -> i_b_m/1
  Manual Switch2/1 -> i_a_m/1
  theta_m/1 -> Manual Switch/2, Sen_pos_r/1(Entrada)
  Manual Switch4/1 -> i_c_m/1
  I_c/1 -> Manual Switch4/2, Sen_c_r/1(Entrada)
  Manual Switch1/1 -> T_s_m/1
  Sen_pos_r/1(Salida) -> Manual Switch/1
  Manual Switch/1 -> theta_m_m/1
  Sen_T_s_r/1(Salida) -> Manual Switch1/1
  Sen_a_r/1(Salida) -> Manual Switch2/1
  Sen_b_r/1(Salida) -> Manual Switch3/1
  Sen_c_r/1(Salida) -> Manual Switch4/1

== system Simulacion_Discretizada/Planta/Subsystem1 ==
  V_a : Inport
  V_b : Inport  Port=2
  V_c : Inport  Port=3
  Inv_a_r : Subsystem
  Inv_b_r : Subsystem
  Inv_c_r : Subsystem
  V_a_s : Outport
  V_b_s : Outport  Port=2
  V_c_s : Outport  Port=3
  wires:
  V_b/1 -> Inv_b_r/1(Entrada)
  Inv_c_r/1(Salida) -> V_c_s/1
  V_c/1 -> Inv_c_r/1(Entrada)
  Inv_b_r/1(Salida) -> V_b_s/1
  V_a/1 -> Inv_a_r/1(Entrada)
  Inv_a_r/1(Salida) -> V_a_s/1

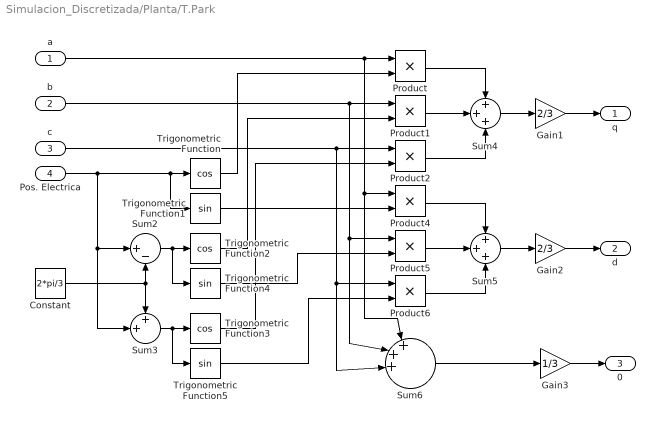
== system Simulacion_Discretizada/Planta/T.Park ==
  a : Inport
  b : Inport  Port=2
  c : Inport  Port=3
  Pos. Electrica : Inport  Port=4
  Constant : Constant  Value=2*pi/3
  Gain1 : Gain  Gain=2/3
  Gain2 : Gain  Gain=2/3
  Gain3 : Gain  Gain=1/3
  Product{,1..2,4..6} (6 alike) : Product
  Sum2 : Sum  Inputs=|+-
  Sum3 : Sum  Inputs=++|
  Sum4 : Sum  Inputs=+++
  Sum5 : Sum  Inputs=+++
  Sum6 : Sum  Inputs=|+|+|+||||
  Trigonometric Function : Trigonometry  Operator=cos
  Trigonometric Function1 : Trigonometry
  Trigonometric Function2 : Trigonometry  Operator=cos
  Trigonometric Function3 : Trigonometry  Operator=cos
  Trigonometric Function4 : Trigonometry
  Trigonometric Function5 : Trigonometry
  q : Outport
  d : Outport  Port=2
  0 : Outport  Port=3
  wires:
  Product1/1 -> Sum4/2
  c/1 -> Product2/1, Product6/1, Sum6/3
  Sum2/1 -> Trigonometric Function4/1, Trigonometric Function2/1
  b/1 -> Product1/1, Product5/1, Sum6/2
  Pos. Electrica/1 -> Trigonometric Function/1, Trigonometric Function1/1, Sum3/2, Sum2/1
  Trigonometric Function2/1 -> Product1/2
  Trigonometric Function5/1 -> Product6/2
  Product6/1 -> Sum5/3
  Trigonometric Function1/1 -> Product4/2
  Constant/1 -> Sum3/1, Sum2/2
  Sum5/1 -> Gain2/1
  Gain1/1 -> q/1
  Sum4/1 -> Gain1/1
  Trigonometric Function3/1 -> Product2/2
  Trigonometric Function/1 -> Product/2
  a/1 -> Product4/1, Sum6/1, Product/1
  Trigonometric Function4/1 -> Product5/2
  Product/1 -> Sum4/1
  Sum3/1 -> Trigonometric Function5/1, Trigonometric Function3/1
  Product2/1 -> Sum4/3
  Product5/1 -> Sum5/2
  Product4/1 -> Sum5/1
  Sum6/1 -> Gain3/1
  Gain3/1 -> 0/1
  Gain2/1 -> d/1

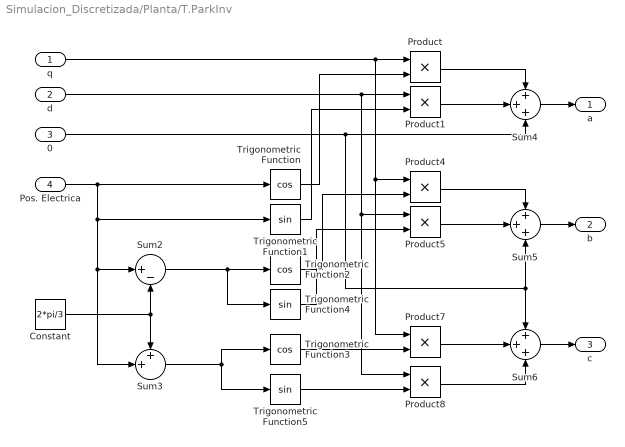
== system Simulacion_Discretizada/Planta/T.ParkInv ==
  q : Inport
  d : Inport  Port=2
  0 : Inport  Port=3
  Pos. Electrica : Inport  Port=4
  Constant : Constant  Value=2*pi/3
  Product{,1,4..5,7..8} (6 alike) : Product
  Sum2 : Sum  Inputs=|+-
  Sum3 : Sum  Inputs=++|
  Sum4 : Sum  Inputs=+++
  Sum5 : Sum  Inputs=+++
  Sum6 : Sum  Inputs=+++
  Trigonometric Function : Trigonometry  Operator=cos
  Trigonometric Function1 : Trigonometry
  Trigonometric Function2 : Trigonometry  Operator=cos
  Trigonometric Function3 : Trigonometry  Operator=cos
  Trigonometric Function4 : Trigonometry
  Trigonometric Function5 : Trigonometry
  a : Outport
  b : Outport  Port=2
  c : Outport  Port=3
  wires:
  Constant/1 -> Sum3/1, Sum2/2
  Pos. Electrica/1 -> Sum3/2, Sum2/1, Trigonometric Function1/1, Trigonometric Function/1
  Trigonometric Function3/1 -> Product7/2
  d/1 -> Product8/1, Product5/1, Product1/1
  0/1 -> Sum6/1, Sum5/3, Sum4/3
  Product8/1 -> Sum6/3
  Product7/1 -> Sum6/2
  q/1 -> Product7/1, Product4/1, Product/1
  Sum3/1 -> Trigonometric Function5/1, Trigonometric Function3/1
  Trigonometric Function5/1 -> Product8/2
  Sum6/1 -> c/1
  Product1/1 -> Sum4/2
  Sum2/1 -> Trigonometric Function4/1, Trigonometric Function2/1
  Sum4/1 -> a/1
  Sum5/1 -> b/1
  Trigonometric Function1/1 -> Product1/2
  Product5/1 -> Sum5/2
  Trigonometric Function2/1 -> Product4/2
  Product4/1 -> Sum5/1
  Product/1 -> Sum4/1
  Trigonometric Function/1 -> Product/2
  Trigonometric Function4/1 -> Product5/2

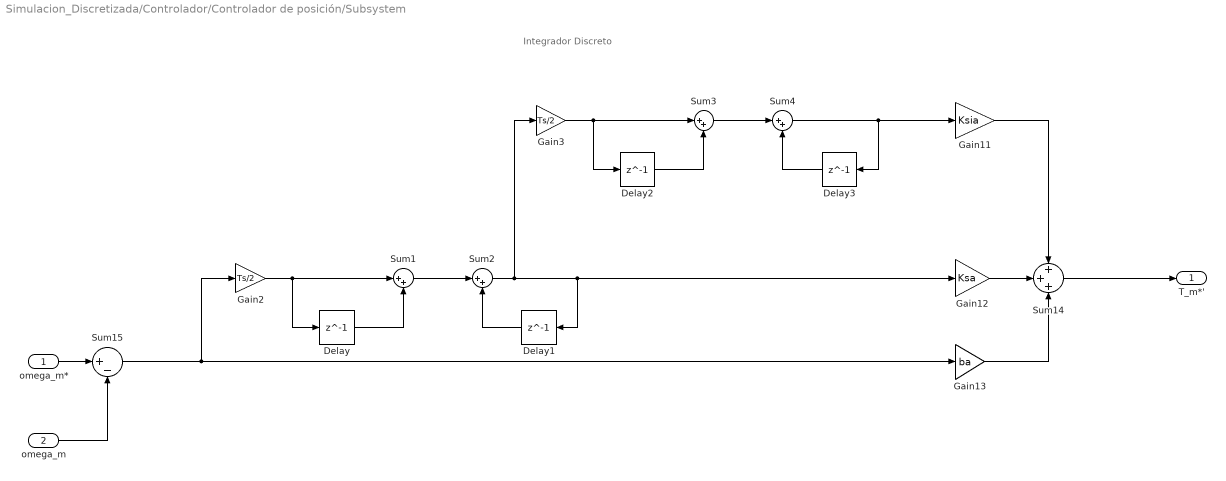
== system Simulacion_Discretizada/Controlador/Controlador de posición/Subsystem ==
  note: Integrador Discreto
  omega_m* : Inport
  omega_m : Inport  Port=2
  Delay{,1..3} (4 alike) : Delay  DelayLength=1  SampleTime=Ts
  Gain11 : Gain  Gain=Ksia
  Gain12 : Gain  Gain=Ksa
  Gain13 : Gain  Gain=ba
  Gain2 : Gain  Gain=Ts/2
  Gain3 : Gain  Gain=Ts/2
  Sum{1..4} (4 alike) : Sum  Inputs=|++
  Sum14 : Sum  Inputs=+++
  Sum15 : Sum  Inputs=|+-
  T_m*' : Outport
  wires:
  Gain12/1 -> Sum14/2
  Sum15/1 -> Gain2/1, Gain13/1
  Delay1/1 -> Sum2/2
  Sum1/1 -> Sum2/1
  Gain11/1 -> Sum14/1
  omega_m*/1 -> Sum15/1
  Sum2/1 -> Gain12/1, Delay1/1, Gain3/1
  Delay2/1 -> Sum3/2
  Delay/1 -> Sum1/2
  Gain13/1 -> Sum14/3
  Sum4/1 -> Gain11/1, Delay3/1
  Gain2/1 -> Sum1/1, Delay/1
  Delay3/1 -> Sum4/2
  Gain3/1 -> Sum3/1, Delay2/1
  Sum3/1 -> Sum4/1
  Sum14/1 -> T_m*'/1
  omega_m/1 -> Sum15/2

== system Simulacion_Discretizada/Controlador/Lazo de control de corrientes/Control de I_ds ==
  note: Linealización por realimentación no lineal
  note: V_ds*'
  i_ds : Inport
  i_qs : Inport  Port=2
  R_s : Inport  Port=3
  omega_e : Inport  Port=4
  i_ds* : Inport  Port=5
  Gain8 : Gain  Gain=Rdp
  Gain9 : Gain  Gain=L_q
  Product1 : Product
  Product3 : Product
  Sum13 : Sum  Inputs=|+-
  Sum7 : Sum  Inputs=||++-
  V_ds* : Outport
  wires:
  i_ds*/1 -> Sum13/1
  Product1/1 -> Sum7/2
  Sum13/1 -> Gain8/1
  Gain9/1 -> Product3/1
  i_ds/1 -> Product1/1, Sum13/2
  Gain8/1 -> Sum7/1
  Product3/1 -> Sum7/3
  omega_e/1 -> Product3/2
  Sum7/1 -> V_ds*/1  "V_ds*"
  i_qs/1 -> Gain9/1
  R_s/1 -> Product1/2

== system Simulacion_Discretizada/Controlador/Lazo de control de corrientes/Control de I_qs ==
  note: V_qs*'
  note: Linealización por realimentación no líneal
  omega_e : Inport
  R_s : Inport  Port=2
  i_ds : Inport  Port=3
  i_qs : Inport  Port=4
  i_qs* : Inport  Port=5
  Constant1 : Constant  Value=lambda_m
  Gain6 : Gain  Gain=Rqp
  Gain7 : Gain  Gain=L_d
  Product2 : Product
  Product4 : Product
  Sum10 : Sum  Inputs=|+-
  Sum8 : Sum  Inputs=||+++
  Sum9 : Sum  Inputs=|++
  V_qs* : Outport
  wires:
  i_qs/1 -> Product2/1, Sum10/2
  Sum10/1 -> Gain6/1
  Product2/1 -> Sum8/2
  omega_e/1 -> Product4/2
  Constant1/1 -> Sum9/1
  Sum9/1 -> Product4/1
  R_s/1 -> Product2/2
  Gain7/1 -> Sum9/2
  Product4/1 -> Sum8/3
  Gain6/1 -> Sum8/1
  i_qs*/1 -> Sum10/1
  Sum8/1 -> V_qs*/1  "V_qs*"
  i_ds/1 -> Gain7/1

== system Simulacion_Discretizada/Controlador/Lazo de control de corrientes/Evolución R_s ==
  T_s : Inport
  Constant1 : Constant  Value=T_sREF
  Constant4 : Constant
  Gain1 : Gain  Gain=alpha_cu
  Gain2 : Gain  Gain=R_sREF
  Sum1 : Sum  Inputs=|+-
  Sum2 : Sum  Inputs=|++
  R_s : Outport
  wires:
  Sum2/1 -> Gain2/1
  Constant4/1 -> Sum2/2
  T_s/1 -> Sum1/1
  Sum1/1 -> Gain1/1
  Gain1/1 -> Sum2/1
  Constant1/1 -> Sum1/2
  Gain2/1 -> R_s/1

== system Simulacion_Discretizada/Controlador/Observador/Int_d ==
  Entrada : Inport
  Delay : Delay  DelayLength=1  SampleTime=Ts
  Delay1 : Delay  DelayLength=1  SampleTime=Ts
  Gain2 : Gain  Gain=Ts/2
  Sum3 : Sum  Inputs=|++
  Sum4 : Sum  Inputs=|++
  Salida : Outport
  wires:
  Delay1/1 -> Sum4/2
  Gain2/1 -> Sum3/1, Delay/1
  Delay/1 -> Sum3/2
  Sum3/1 -> Sum4/1
  Sum4/1 -> Salida/1, Delay1/1
  Entrada/1 -> Gain2/1

== system Simulacion_Discretizada/Controlador/Observador/Int_d1 ==
  Entrada : Inport
  Delay : Delay  DelayLength=1  SampleTime=Ts
  Delay1 : Delay  DelayLength=1  SampleTime=Ts
  Gain2 : Gain  Gain=Ts/2
  Sum3 : Sum  Inputs=|++
  Sum4 : Sum  Inputs=|++
  Salida : Outport
  wires:
  Delay1/1 -> Sum4/2
  Gain2/1 -> Sum3/1, Delay/1
  Delay/1 -> Sum3/2
  Sum3/1 -> Sum4/1
  Sum4/1 -> Salida/1, Delay1/1
  Entrada/1 -> Gain2/1

== system Simulacion_Discretizada/Controlador/Observador/Int_d2 ==
  Entrada : Inport
  Delay : Delay  DelayLength=1  SampleTime=Ts
  Delay1 : Delay  DelayLength=1  SampleTime=Ts
  Gain2 : Gain  Gain=Ts/2
  Sum3 : Sum  Inputs=|++
  Sum4 : Sum  Inputs=|++
  Salida : Outport
  wires:
  Delay1/1 -> Sum4/2
  Gain2/1 -> Sum3/1, Delay/1
  Delay/1 -> Sum3/2
  Sum3/1 -> Sum4/1
  Sum4/1 -> Salida/1, Delay1/1
  Entrada/1 -> Gain2/1

== system Simulacion_Discretizada/Controlador/Observador/Int_d3 ==
  Entrada : Inport
  Delay : Delay  DelayLength=1  SampleTime=Ts
  Delay1 : Delay  DelayLength=1  SampleTime=Ts
  Gain2 : Gain  Gain=Ts/2
  Sum3 : Sum  Inputs=|++
  Sum4 : Sum  Inputs=|++
  Salida : Outport
  wires:
  Delay1/1 -> Sum4/2
  Gain2/1 -> Sum3/1, Delay/1
  Delay/1 -> Sum3/2
  Sum3/1 -> Sum4/1
  Sum4/1 -> Salida/1, Delay1/1
  Entrada/1 -> Gain2/1

== system Simulacion_Discretizada/Planta/Subsistema electromagnético/Subsystem ==
  V_qs : Inport
  R_s : Inport  Port=2
  omega_e : Inport  Port=3
  i_ds*L_d : Inport  Port=4
  Constant : Constant  Value=lambda_m
  Gain8 : Gain  Gain=1/L_q
  Integrator3 : Integrator
  Product : Product
  Product5 : Product
  Sum3 : Sum  Inputs=||+--
  Sum4 : Sum  Inputs=|++
  i_qs : Outport
  wires:
  Constant/1 -> Sum4/2
  Product5/1 -> Sum3/3
  V_qs/1 -> Sum3/1
  i_ds*L_d/1 -> Sum4/1
  Product/1 -> Sum3/2
  Gain8/1 -> Integrator3/1
  Integrator3/1 -> Product5/1, i_qs/1  "i_qs"
  Sum4/1 -> Product/2
  Sum3/1 -> Gain8/1
  R_s/1 -> Product5/2
  omega_e/1 -> Product/1

== system Simulacion_Discretizada/Planta/Subsistema electromagnético/Subsystem1 ==
  i_qs*Lq : Inport
  omega_e : Inport  Port=2
  R_s : Inport  Port=3
  V_ds : Inport  Port=4
  Gain : Gain  Gain=1/L_d
  Integrator4 : Integrator
  Product10 : Product
  Product2 : Product
  Sum5 : Sum  Inputs=||++-
  i_ds : Outport
  wires:
  Product10/1 -> Sum5/3
  i_qs*Lq/1 -> Product2/1
  Gain/1 -> Integrator4/1
  V_ds/1 -> Sum5/1
  Sum5/1 -> Gain/1
  R_s/1 -> Product10/2
  Product2/1 -> Sum5/2
  omega_e/1 -> Product2/2
  Integrator4/1 -> i_ds/1, Product10/1  "i_ds"

== system Simulacion_Discretizada/Planta/Subsistema electromagnético/Subsystem2 ==
  R_s : Inport
  V_0s : Inport  Port=2
  Gain1 : Gain  Gain=1/L_ls
  Integrator5 : Integrator
  Product11 : Product
  Sum6 : Sum  Inputs=|+-
  i_0s : Outport
  wires:
  Integrator5/1 -> i_0s/1, Product11/1  "i_0s"
  Product11/1 -> Sum6/2
  R_s/1 -> Product11/2
  Sum6/1 -> Gain1/1
  Gain1/1 -> Integrator5/1
  V_0s/1 -> Sum6/1

== system Simulacion_Discretizada/Planta/Subsistema electromagnético/Subsystem3 ==
  I_ds : Inport
  i_qs : Inport  Port=2
  Gain5 : Gain  Gain=L_d-L_q
  Gain6 : Gain  Gain=3*P_p/2
  Gain7 : Gain  Gain=lambda_m
  Product1 : Product
  Sum2 : Sum  Inputs=|++
  T_m : Outport
  wires:
  Sum2/1 -> Gain6/1
  Gain7/1 -> Sum2/1
  I_ds/1 -> Product1/2
  Gain5/1 -> Sum2/2
  i_qs/1 -> Product1/1, Gain7/1
  Gain6/1 -> T_m/1
  Product1/1 -> Gain5/1

== system Simulacion_Discretizada/Planta/Subsystem/Sen_T_s_r ==
  Entrada : Inport
  Gain1 : Gain  Gain=1/tau
  Gain3 : Gain  Gain=1/tau
  Integrator : Integrator  InitialCondition=T_amb
  Sum : Sum  Inputs=|+-
  Salida : Outport
  wires:
  Sum/1 -> Integrator/1
  Integrator/1 -> Gain1/1, Salida/1
  Gain3/1 -> Sum/1
  Entrada/1 -> Gain3/1
  Gain1/1 -> Sum/2

== system Simulacion_Discretizada/Planta/Subsystem/Sen_a_r ==
  Entrada : Inport
  2.zit.omega_n^2 : Gain  Gain=2*zit_i*w_n_i
  Integrator : Integrator
  Integrator1 : Integrator
  Sum : Sum  Inputs=|+--
  omega_n^2 : Gain  Gain=w_n_i^2
  omega_n^2_2 : Gain  Gain=w_n_i^2
  Salida : Outport
  wires:
  Integrator1/1 -> 2.zit.omega_n^2/1, Integrator/1
  Integrator/1 -> Salida/1, omega_n^2_2/1
  omega_n^2_2/1 -> Sum/2
  omega_n^2/1 -> Sum/1
  Sum/1 -> Integrator1/1
  Entrada/1 -> omega_n^2/1
  2.zit.omega_n^2/1 -> Sum/3

== system Simulacion_Discretizada/Planta/Subsystem/Sen_b_r ==
  Entrada : Inport
  Gain1 : Gain  Gain=2*zit_i*w_n_i
  Gain2 : Gain  Gain=w_n_i^2
  Gain3 : Gain  Gain=w_n_i^2
  Integrator : Integrator
  Integrator1 : Integrator
  Sum : Sum  Inputs=|+--
  Salida : Outport
  wires:
  Integrator1/1 -> Gain1/1, Integrator/1
  Integrator/1 -> Salida/1, Gain2/1
  Gain2/1 -> Sum/2
  Gain3/1 -> Sum/1
  Sum/1 -> Integrator1/1
  Entrada/1 -> Gain3/1
  Gain1/1 -> Sum/3

== system Simulacion_Discretizada/Planta/Subsystem/Sen_c_r ==
  Entrada : Inport
  Gain1 : Gain  Gain=2*zit_i*w_n_i
  Gain2 : Gain  Gain=w_n_i^2
  Gain3 : Gain  Gain=w_n_i^2
  Integrator : Integrator
  Integrator1 : Integrator
  Sum : Sum  Inputs=|+--
  Salida : Outport
  wires:
  Integrator1/1 -> Gain1/1, Integrator/1
  Integrator/1 -> Salida/1, Gain2/1
  Gain2/1 -> Sum/2
  Gain3/1 -> Sum/1
  Sum/1 -> Integrator1/1
  Entrada/1 -> Gain3/1
  Gain1/1 -> Sum/3

== system Simulacion_Discretizada/Planta/Subsystem/Sen_pos_r ==
  Entrada : Inport
  Gain1 : Gain  Gain=2*zit_pos*w_n_pos
  Gain2 : Gain  Gain=w_n_pos^2
  Gain3 : Gain  Gain=w_n_pos^2
  Integrator : Integrator
  Integrator1 : Integrator
  Sum : Sum  Inputs=|+--
  Salida : Outport
  wires:
  Integrator1/1 -> Gain1/1, Integrator/1
  Integrator/1 -> Salida/1, Gain2/1
  Gain2/1 -> Sum/2
  Gain3/1 -> Sum/1
  Sum/1 -> Integrator1/1
  Entrada/1 -> Gain3/1
  Gain1/1 -> Sum/3

== system Simulacion_Discretizada/Planta/Subsystem1/Inv_a_r ==
  Entrada : Inport
  2.zit.omega_n^2 : Gain  Gain=2*zit_v*w_n_v
  Integrator : Integrator
  Integrator1 : Integrator
  Saturation : Saturate  UpperLimit=V_max  LowerLimit=-V_max
  Sum : Sum  Inputs=|+--
  omega_n^2 : Gain  Gain=w_n_v^2
  omega_n^2_2 : Gain  Gain=w_n_v^2
  Salida : Outport
  wires:
  Integrator1/1 -> 2.zit.omega_n^2/1, Integrator/1
  Integrator/1 -> Salida/1, omega_n^2_2/1
  omega_n^2_2/1 -> Sum/2
  omega_n^2/1 -> Sum/1
  Sum/1 -> Integrator1/1
  Entrada/1 -> Saturation/1
  2.zit.omega_n^2/1 -> Sum/3
  Saturation/1 -> omega_n^2/1

== system Simulacion_Discretizada/Planta/Subsystem1/Inv_b_r ==
  Entrada : Inport
  2.zit.omega_n^2 : Gain  Gain=2*zit_v*w_n_v
  Integrator : Integrator
  Integrator1 : Integrator
  Saturation : Saturate  UpperLimit=V_max  LowerLimit=-V_max
  Sum : Sum  Inputs=|+--
  omega_n^2 : Gain  Gain=w_n_v^2
  omega_n^2_2 : Gain  Gain=w_n_v^2
  Salida : Outport
  wires:
  Integrator1/1 -> 2.zit.omega_n^2/1, Integrator/1
  Integrator/1 -> Salida/1, omega_n^2_2/1
  omega_n^2_2/1 -> Sum/2
  omega_n^2/1 -> Sum/1
  Sum/1 -> Integrator1/1
  Entrada/1 -> Saturation/1
  2.zit.omega_n^2/1 -> Sum/3
  Saturation/1 -> omega_n^2/1

== system Simulacion_Discretizada/Planta/Subsystem1/Inv_c_r ==
  Entrada : Inport
  2.zit.omega_n^2 : Gain  Gain=2*zit_v*w_n_v
  Integrator : Integrator
  Integrator1 : Integrator
  Saturation : Saturate  UpperLimit=V_max  LowerLimit=-V_max
  Sum : Sum  Inputs=|+--
  omega_n^2 : Gain  Gain=w_n_v^2
  omega_n^2_2 : Gain  Gain=w_n_v^2
  Salida : Outport
  wires:
  Integrator1/1 -> 2.zit.omega_n^2/1, Integrator/1
  Integrator/1 -> Salida/1, omega_n^2_2/1
  omega_n^2_2/1 -> Sum/2
  omega_n^2/1 -> Sum/1
  Sum/1 -> Integrator1/1
  Entrada/1 -> Saturation/1
  2.zit.omega_n^2/1 -> Sum/3
  Saturation/1 -> omega_n^2/1

== matlab function Simulacion_Discretizada/MATLAB Function ==
  data: t input; y output; sol input; sol2 input
function y = fcn(t,sol,sol2)
if (t>= 1) && (t< 6)
    y = sol(1)*t^5 + sol(2)*t^4 + sol(3)*t^3 + sol(4)*t^2 + sol(5)*t + sol(6);
elseif (t>= 6) && (t< 11)
    y = 2*pi;
elseif (t>= 11) && (t<= 16)
    y = sol2(1)*t^5 + sol2(2)*t^4 + sol2(3)*t^3 + sol2(4)*t^2 + sol2(5)*t + sol2(6);
else
    y = 0;
end
end

== matlab function Simulacion_Discretizada/Controlador/Controlador de posición/consigna_velocidad ==
  data: t input; y output; sol input; sol2 input
function y = fcn(t,sol,sol2)
if (t>= 1) && (t< 6)
    y = 5*sol(1)*t^4 + 4*sol(2)*t^3 + 3*sol(3)*t^2 + 2*sol(4)*t + sol(5);
elseif (t>= 6) && (t< 11)
    y = 0;
elseif (t>= 11) && (t<= 16)
    y = 5*sol2(1)*t^4 + 4*sol2(2)*t^3 + 3*sol2(3)*t^2 + 2*sol2(4)*t + sol2(5);
else
    y = 0;
end
end
